simulink model "statechart"  (R2016b)
settings: Solver=VariableStepAuto  StartTime=0.0  StopTime=6.5  MaxStep=0.05  RelTol=1e-3
libraries: dspindex x3
settings Model: Creator=larry  LastModifiedBy=larry

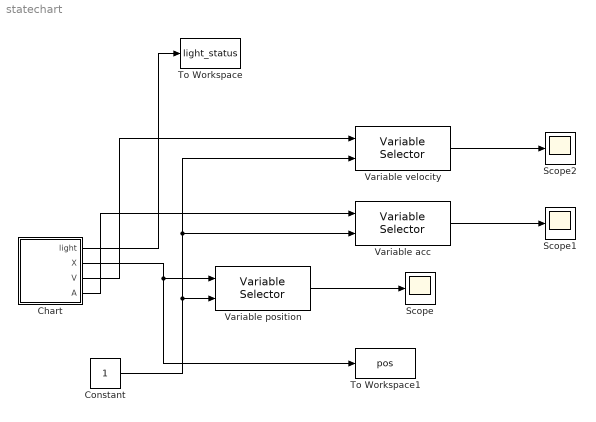
== system statechart ==
  Chart : Stateflow chart  TreatAsAtomicUnit=on
  Constant : Constant
  Scope : Scope
  Scope1 : Scope
  Scope2 : Scope
  To Workspace : ToWorkspace  VariableName=light_status  SampleTime=-1
  To Workspace1 : ToWorkspace  VariableName=pos  SampleTime=-1
  Variable acc : dspindex/Variable Selector  NumInputs=1  rowsOrCols=Columns  IdxMode=Variable  Elements=[1 3]  ZerOneIdxMode=One-based  errmode=Clip Index  FillMode=on  FillValues=0
  Variable position : dspindex/Variable Selector  NumInputs=1  rowsOrCols=Columns  IdxMode=Variable  Elements=[1 3]  ZerOneIdxMode=One-based  errmode=Clip Index  FillMode=on  FillValues=0
  Variable velocity : dspindex/Variable Selector  NumInputs=1  rowsOrCols=Columns  IdxMode=Variable  Elements=[1 3]  ZerOneIdxMode=One-based  errmode=Clip Index  FillMode=on  FillValues=0
  wires:
  Chart/1(light) -> To Workspace/1
  Chart/2(X) -> To Workspace1/1, Variable position/1
  Constant/1 -> Variable acc/2, Variable velocity/2, Variable position/2
  Variable position/1 -> Scope/1
  Variable acc/1 -> Scope1/1
  Variable velocity/1 -> Scope2/1
  Chart/3(V) -> Variable velocity/1
  Chart/4(A) -> Variable acc/1

== stateflow chart statechart/Chart ==
  state Light [parallel]
    settings: executionOrder=1
    state RED
      en:
      light = 1;
    state GREEN
      en:
      light = 0;
    (default) -> RED
    RED -> GREEN : after(2.5, sec)
    GREEN -> RED : after(2.5, sec)
  state Vehicle1 [parallel]
    settings: executionOrder=2
    state Straight
      state FreeDriving
        state AccFromStop
          en:
          A(this,:) = [A_MAX, 0];
          du:
          [X(this,:), V(this,:)] = accDrive(this, X, V, A);
        state Acc
          en:
          A(this,:) = [0.5*A_MAX, 0];
          du:
          [X(this,:), V(this,:)] = accDrive(this, X, V, A);
        state FixRate
          en:
          A(this,:) = [0, 0];
          V(this,:) = fixRate(this, V, V_MAX);
          du:
          X(this,:) = fixRateDrive(this, X, V);
        (default) -> (junction 71)
        (junction 71) -> Vehicle1.Straight.FreeDriving.AccFromStop [order 2]
        (junction 71) -> (junction 299) [order 1] : [~isStopped(this, V, D)]
        Vehicle1.Straight.FreeDriving.AccFromStop -> Vehicle1.Straight.FreeDriving.Acc : [reach(this, V, 3.0/5*V_MAX)]
        (junction 299) -> Vehicle1.Straight.FreeDriving.Acc [order 2]
        (junction 299) -> Vehicle1.Straight.FreeDriving.FixRate [order 1] : [reach(this, V, V_MAX)]
        Vehicle1.Straight.FreeDriving.Acc -> Vehicle1.Straight.FreeDriving.FixRate : [reach(this, V, V_MAX)]
      state Follow
        du:
        [X(this,:), V(this,:), A(this,:)] = ...
        followFrontCar(this, X, V, D, A_MAX);
      (default) -> Vehicle1.Straight.FreeDriving
      Vehicle1.Straight.FreeDriving -> Vehicle1.Straight.Follow : [hasFrontCar(this, X, D)]
      Vehicle1.Straight.Follow -> Vehicle1.Straight.FreeDriving : [~hasFrontCar(this, X, D)]
    state SlowToStop
      state SlowDown
        en:
        A(this,:) = reqAcc(this, X, V, A_MAX, stop);
        du:
        [X(this,:), V(this,:)] = accDrive(this, X, V, A);
      state Stopped
        en:
        A(this,:) = [0, 0];
        V(this,:) = [0, 0];
      (default) -> Vehicle1.SlowToStop.SlowDown
      Vehicle1.SlowToStop.SlowDown -> Vehicle1.SlowToStop.Stopped : [isStopped(this, V, D)]
    (default) -> Vehicle1.Straight
    Vehicle1.SlowToStop -> Vehicle1.Straight : [in(Light.GREEN)]
    (junction 1589) -> Vehicle1.SlowToStop
    (junction 1588) -> (junction 1589) [order 1] : [hasFrontCar(this, X, D)]...
        | {stop = getStopPos(this, X, D, INTER)
        | X(this,:)
        | X(2,:)}
    Vehicle1.Straight -> (junction 1588) : [in(Light.RED) &&...
        | closeToInter(this,X,D,INTER)]
    (junction 1590) -> (junction 1589) [order 1] : [isStoppable(this,X,V,A_MAX,INTER)]...
        | {stop = INTER}
    (junction 1588) -> (junction 1590) [order 2]
    (junction 1590) -> Vehicle1.Straight [order 2]
  state Vehicle2 [parallel]
    settings: executionOrder=3
    state Straight
      state FreeDriving
        state AccFromStop
          en:
          A(this,:) = [A_MAX, 0];
          du:
          [X(this,:), V(this,:)] = accDrive(this, X, V, A);
        state Acc
          en:
          A(this,:) = [0.5*A_MAX, 0];
          du:
          [X(this,:), V(this,:)] = accDrive(this, X, V, A);
        state FixRate
          en:
          A(this,:) = [0, 0];
          V(this,:) = fixRate(this, V, V_MAX);
          du:
          X(this,:) = fixRateDrive(this, X, V);
        (default) -> (junction 1905)
        (junction 1905) -> Vehicle2.Straight.FreeDriving.AccFromStop [order 2]
        (junction 1905) -> (junction 1906) [order 1] : [~isStopped(this, V, D)]
        Vehicle2.Straight.FreeDriving.AccFromStop -> Vehicle2.Straight.FreeDriving.Acc : [reach(this, V, 3.0/5*V_MAX)]
        (junction 1906) -> Vehicle2.Straight.FreeDriving.Acc [order 2]
        (junction 1906) -> Vehicle2.Straight.FreeDriving.FixRate [order 1] : [reach(this, V, V_MAX)]
        Vehicle2.Straight.FreeDriving.Acc -> Vehicle2.Straight.FreeDriving.FixRate : [reach(this, V, V_MAX)]
      state Follow
        du:
        [X(this,:), V(this,:), A(this,:)] = ...
        followFrontCar(this, X, V, D, A_MAX);
      (default) -> Vehicle2.Straight.FreeDriving
      Vehicle2.Straight.FreeDriving -> Vehicle2.Straight.Follow : [hasFrontCar(this, X, D)]
      Vehicle2.Straight.Follow -> Vehicle2.Straight.FreeDriving : [~hasFrontCar(this, X, D)]
    state SlowToStop
      state SlowDown
        en:
        A(this,:) = reqAcc(this, X, V, A_MAX, stop);
        du:
        [X(this,:), V(this,:)] = accDrive(this, X, V, A);
      state Stopped
        en:
        A(this,:) = [0, 0];
        V(this,:) = [0, 0];
      (default) -> Vehicle2.SlowToStop.SlowDown
      Vehicle2.SlowToStop.SlowDown -> Vehicle2.SlowToStop.Stopped : [isStopped(this, V, D)]
    (default) -> Vehicle2.Straight
    Vehicle2.SlowToStop -> Vehicle2.Straight : [in(Light.GREEN)]
    (junction 1889) -> Vehicle2.SlowToStop
    (junction 1890) -> (junction 1889) [order 1] : [hasFrontCar(this, X, D)]...
        | {stop = getStopPos(this, X, D, INTER);}
    Vehicle2.Straight -> (junction 1890) : [in(Light.RED) &&...
        | closeToInter(this,X,D,INTER)]
    (junction 1891) -> (junction 1889) [order 1] : [isStoppable(this,X,V,A_MAX,INTER)]...
        | {stop = INTER;}
    (junction 1890) -> (junction 1891) [order 2]
    (junction 1891) -> Vehicle2.Straight [order 2]
  state Vehicle3 [parallel]
    settings: executionOrder=4
    state Straight
      state FreeDriving
        state AccFromStop
          en:
          A(this,:) = [A_MAX, 0];
          du:
          [X(this,:), V(this,:)] = accDrive(this, X, V, A);
        state Acc
          en:
          A(this,:) = [0.5*A_MAX, 0];
          du:
          [X(this,:), V(this,:)] = accDrive(this, X, V, A);
        state FixRate
          en:
          A(this,:) = [0, 0];
          V(this,:) = fixRate(this, V, V_MAX);
          du:
          X(this,:) = fixRateDrive(this, X, V);
        (default) -> (junction 1945)
        (junction 1945) -> Vehicle3.Straight.FreeDriving.AccFromStop [order 2]
        (junction 1945) -> (junction 1946) [order 1] : [~isStopped(this, V, D)]
        Vehicle3.Straight.FreeDriving.AccFromStop -> Vehicle3.Straight.FreeDriving.Acc : [reach(this, V, 3.0/5*V_MAX)]
        (junction 1946) -> Vehicle3.Straight.FreeDriving.Acc [order 2]
        (junction 1946) -> Vehicle3.Straight.FreeDriving.FixRate [order 1] : [reach(this, V, V_MAX)]
        Vehicle3.Straight.FreeDriving.Acc -> Vehicle3.Straight.FreeDriving.FixRate : [reach(this, V, V_MAX)]
      state Follow
        du:
        [X(this,:), V(this,:), A(this,:)] = ...
        followFrontCar(this, X, V, D, A_MAX);
      (default) -> Vehicle3.Straight.FreeDriving
      Vehicle3.Straight.FreeDriving -> Vehicle3.Straight.Follow : [hasFrontCar(this, X, D)]
      Vehicle3.Straight.Follow -> Vehicle3.Straight.FreeDriving : [~hasFrontCar(this, X, D)]
    state SlowToStop
      state SlowDown
        en:
        A(this,:) = reqAcc(this, X, V, A_MAX, stop);
        du:
        [X(this,:), V(this,:)] = accDrive(this, X, V, A);
      state Stopped
        en:
        A(this,:) = [0, 0];
        V(this,:) = [0, 0];
      (default) -> Vehicle3.SlowToStop.SlowDown
      Vehicle3.SlowToStop.SlowDown -> Vehicle3.SlowToStop.Stopped : [isStopped(this, V, D)]
    (default) -> Vehicle3.Straight
    Vehicle3.SlowToStop -> Vehicle3.Straight : [in(Light.GREEN)]
    (junction 1929) -> Vehicle3.SlowToStop
    (junction 1930) -> (junction 1929) [order 1] : [hasFrontCar(this, X, D)]...
        | {stop = getStopPos(this, X, D, INTER);}
    Vehicle3.Straight -> (junction 1930) : [in(Light.RED) &&...
        | closeToInter(this,X,D,INTER)]
    (junction 1931) -> (junction 1929) [order 1] : [isStoppable(this,X,V,A_MAX,INTER)]...
        | {stop = INTER;}
    (junction 1930) -> (junction 1931) [order 2]
    (junction 1931) -> Vehicle3.Straight [order 2]
  data: self function_input; Xi function_input; Vi function_input; amax function_input; a function_output; inter function_input; self function_input; Vi function_input; Di function_input; res function_output; self function_input; res function_output; Xi function_input; Di function_input; self function_input; Xi function_input; Vi function_input; x function_output; self function_input; res function_output; Xi function_input; Di function_input; inter function_input; self function_input; Vi function_input; s function_input; v function_output; self function_input; Xi function_input; Vi function_input; Ai function_input; x function_output; v function_output; this constant uint8 size=1 =1; V_MAX constant double size=1 =2.5; A_MAX constant double size=1 =2.5; stop local double size=[1, 2] =[0, 0]; INTER local double size=[1, 2] =[-1, -0.5]; this constant uint8 size=1 =2; V_MAX constant double size=1 =2.5; A_MAX constant double size=1 =2.5; stop local double size=[1, 2] =[0, 0]; INTER local double size=[1, 2] =[-1, -0.5]; self function_input; res function_output; Xi function_input; Vi function_input; Di function_input; amax function_input; inter function_input; self function_input; Xi function_input; Vi function_input; amax function_input; res function_output; inter function_input; this constant uint8 size=1 =3; V_MAX constant double size=1 =2.5; A_MAX constant double size=1 =2.5; stop local double size=[1, 2] =[0, 0]; INTER local double size=[1, 2] =[-1, -0.5]; self function_input; Vi function_input; vmax function_input; res function_output; self function_input; Xi function_input; Vi function_input; Di function_input; x function_output; v function_output; amax function_input; a function_output; self function_input; Xi function_input; pos function_output; Di function_input; inter function_input; dt constant double size=1 =0.05; light output size=1; WORLD_SIZE constant double size=1 =8; X output size=[3,2] =[5 -0.5;7 -0.5;-5 -0.5]; D local size=[3,2] =[1 0;1 0;1 0]; SAFE_DIST constant double size=1 =1; V output size=[3,2] =[0 0;0 0;0 0]; A output size=[3,2] =[0 0;0 0;0 0]
  function a = reqAcc(self, Xi, Vi, amax, inter):
    | function a = reqAcc(self, Xi, Vi, amax, inter)
    | 
    | x = Xi(self, :);
    | v = Vi(self, :);
    | 
    | dx = inter - x;
    | % add safe distance
    | dist = norm(dx) - SAFE_DIST;
    | if dot(dx, v) < 0
    |     a = [0 0];
    | else
    |     vnorm = norm(v);
    |     reverse = v/vnorm*(-1);
    |     a = reverse*vnorm*vnorm/2/dist;
    |     anorm = norm(a);
    |     if(anorm >= amax)
    |         a = a/anorm*amax;
    |     end
    | end
  function res = isStopped(self, Vi, Di):
    | function res = isStopped(self, Vi, Di)
    | 
    | v = Vi(self,:);
    | d = Di(self,:);
    | res = false;
    | if(dot(v, d) <= 0)
    |     res = true;
    | end
    | if norm(v) <= 1e-3
    |     res = true;
    | end
  function res = hasFrontCar(self, Xi, Di):
    | function res = hasFrontCar(self, Xi, Di)
    | 
    | res = false;
    | num = size(Xi, 1);
    | if num == 1
    |     return;
    | end
    | 
    | dX = zeros(num, 1);
    | x = Xi(self,:);
    | d = Di(self,:);
    | for k=1:length(dX)
    |     dX(k) = dot(Xi(k,:) - x, d);
    |     if dX(k) < 0
    |         dX(k) = dX(k) + 2*WORLD_SIZE;
    |     end
    | end
    | 
    | % set zero dX to a large enough value
    | dX(dX == 0) = 100;
    | close = min(dX);
    | if close <= 2*SAFE_DIST
    |     res = true;
    | end
  function x = fixRateDrive(self, Xi, Vi):
    | function x = fixRateDrive(self, Xi, Vi)
    |  
    | x = Xi(self, :);
    | v = Vi(self, :);
    | 
    | x = x + v * dt;
    | 
    | % a rounded world
    | if x(1) > WORLD_SIZE
    |     x(1) = -WORLD_SIZE;
    | elseif x(1) < -WORLD_SIZE
    |     x(1) = WORLD_SIZE;
    | end
  function res = closeToInter(self, Xi, Di, inter):
    | function res = closeToInter(self, Xi, Di, inter)
    | 
    | x = Xi(self, :);
    | d = Di(self, :);
    | 
    | inner = dot(inter - x, d);
    | if inner >= 0 && inner <= 2.5
    |     res = true;
    | else
    |     res = false;
    | end
  function v = fixRate(self, Vi, s):
    | function v = fixRate(self, Vi, s)
    |  
    | v = Vi(self, :);
    | if norm(v) < 1e-6
    |     v = [0 0];
    | else
    |     v = v/norm(v)*s;
    | end
  function [x, v] = accDrive(self, Xi, Vi, Ai):
    | function [x, v] = accDrive(self, Xi, Vi, Ai)
    | 
    | x = Xi(self, :);
    | v = Vi(self, :);
    | a = Ai(self, :);
    | 
    | x = x + v * dt + 0.5 * a * dt * dt;
    | v = v + a * dt;
    | 
    | if x(1) > WORLD_SIZE
    |     x(1) = -WORLD_SIZE;
    | elseif x(1) < -WORLD_SIZE
    |     x(1) = WORLD_SIZE;
    | end
  function res = stoppedByRed(self, Xi, Vi, Di, amax, inter):
    | function res = stoppedByRed(self, Xi, Vi, Di, amax, inter)
    | 
    | if closeToInter(self, Xi, Di, inter) && ...
    |         isStoppable(self, Xi, Vi, amax, inter) && ...
    |         in(Light.RED)
    |     res = true;
    | else
    |     res = false;
    | end
  function res = isStoppable(self, Xi, Vi, amax, inter):
    | function res = isStoppable(self, Xi, Vi, amax, inter)
    | 
    | x = Xi(self, :);
    | v = Vi(self, :);
    | dist = norm(inter - x);
    | 
    | vnorm = norm(v);
    | brake_dist = vnorm*vnorm/2.0/amax;
    | res = (brake_dist <= dist);
  function res = reach(self, Vi, vmax):
    | function res = reach(self, Vi, vmax)
    | 
    | res = false;
    | if norm(Vi(self, :)) >= vmax
    |     res = true;
    | end
  function [x, v, a] = followFrontCar(self, Xi, Vi, Di, amax):
    | function [x, v, a] = followFrontCar(self, Xi, Vi, Di, amax)
    | 
    | dX = zeros(size(Xi, 1), 1);
    | x = Xi(self,:);
    | v = Vi(self,:);
    | d = Di(self,:);
    | a = [0, 0];
    | 
    | for k=1:length(dX)
    |     dX(k) = dot(Xi(k,:) - x, d);
    |     if dX(k) < 0
    |         dX(k) = dX(k) + 2*WORLD_SIZE;
    |     end
    | end
    | 
    | % set zero dX to a large enough value
    | dX(dX == 0) = 100;
    | [dist, idx] = min(dX);
    | 
    | % % idx = find(dX == dist);
    | 
    | % there must be only one vehicle in front of target agent
    | assert(length(idx) == 1);
    | vo = Vi(idx(1), :);
    | 
    | if dist < 2*SAFE_DIST
    |     
    |     if dist <= 1.5*SAFE_DIST
    |         vo = 0.75*vo;
    |     elseif dist <= SAFE_DIST
    |         vo = 0.5*vo;
    |     end
    |     
    |     ar = (vo - v) / dt;
    |     arnorm = norm(ar);
    |     if arnorm > amax
    |         ar = ar/arnorm * amax;
    |         x = x + v * dt + 0.5 * ar * dt * dt;
    |         v = v + ar * dt;
    |     else
    |         x = x + (v + vo) * dt / 2;
    |         v = vo;
    |     end
    |     a = ar;
    | end
    | 
    | % a rounded world
    | if x(1) > WORLD_SIZE
    |     x(1) = -WORLD_SIZE;
    | elseif x(1) < -WORLD_SIZE
    |     x(1) = WORLD_SIZE;
    | end
  function pos = getStopPos(self, Xi, Di, inter):
    | function pos = getStopPos(self, Xi, Di, inter)
    | 
    | dX = zeros(size(Xi, 1), 1);
    | x = Xi(self,:);
    | d = Di(self,:);
    | 
    | for k=1:length(dX)
    |     dX(k) = dot(Xi(k,:) - x, d);
    |     if dX(k) < 0
    |         dX(k) = dX(k) + 2*WORLD_SIZE;
    |     end
    | end
    | 
    | % set zero dX to a large enough value
    | dX(dX == 0) = 100;
    | [frontDist, index] = min(dX);
    | interDist = dot(inter - x, d);
    | 
    | if frontDist < interDist
    |     pos = Xi(index,:);
    | else
    |     pos = inter;
    | end
